simulink model "simulacao_relatorio"  (R2018a)
settings: Solver=VariableStepAuto  StartTime=0.0  StopTime=10000  RelTol=1e-3
undefined symbols (not defined in the file or in its folder): sigbuilder_block
settings Model: Creator=Christopher  LastModifiedBy=Christopher

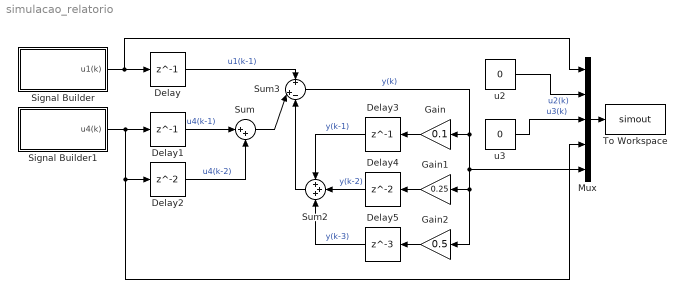
== system simulacao_relatorio ==
  Delay : Delay  DelayLength=1
  Delay1 : Delay  DelayLength=1
  Delay2 : Delay
  Delay3 : Delay  DelayLength=1
  Delay4 : Delay
  Delay5 : Delay  DelayLength=3
  Gain : Gain  Gain=0.1
  Gain1 : Gain  Gain=0.25
  Gain2 : Gain  Gain=0.5
  Mux : Mux  Inputs=5
  Signal Builder : Subsystem  Tag=STV Subsys  LoadFcn=sigbuilder_block('load',[437.6 199.2 550.4 400 ]);  StartFcn=sigbuilder_block('start');  StopFcn=sigbuilder_block('stop');  ClipboardFcn=sigbuilder_block('clipboard');  mask(Sigbuilder block){tuvar=[0:10]}
      mask help: Simulink:masks:SigbuilderBlock_MD
      mask init:
      | if ~strcmp(get_param(bdroot(gcbh),'SimulationStatus'),'stopped') tuvar = sigbuilder_block('maskInit'); end
      settings: CopyFcn=sigbuilder_block('copy');  DeleteFcn=sigbuilder_block('delete');  ModelCloseFcn=sigbuilder_block('modelClose');  PreSaveFcn=sigbuilder_block('preSave');  PauseFcn=sigbuilder_block('pause');  ContinueFcn=sigbuilder_block('continue');  NameChangeFcn=sigbuilder_block('namechange');  OpenFcn=sigbuilder_block('open',[437.6 199.2 550.4 400 ]);  CloseFcn=sigbuilder_block('close');
      mask Display: plot(0, 0, 100, 100,[2, 2, 32, 32, 2], [68, 8, 8, 68, 68],[32, 2], [38, 38], [32, 19, 2],[53, 60, 44], [32, 17, 17, 2],[16, 16, 31, 31]);txt = getActiveGroup(gcbh);text(2, 100, txt,'verticalAlignment', 'top');
  Signal Builder1 : Subsystem  Tag=STV Subsys  LoadFcn=sigbuilder_block('load');  StartFcn=sigbuilder_block('start');  StopFcn=sigbuilder_block('stop');  ClipboardFcn=sigbuilder_block('clipboard');  mask(Sigbuilder block){tuvar=[0:10]}
      mask help: Simulink:masks:SigbuilderBlock_MD
      mask init:
      | if ~strcmp(get_param(bdroot(gcbh),'SimulationStatus'),'stopped') tuvar = sigbuilder_block('maskInit'); end
      settings: CopyFcn=sigbuilder_block('copy');  DeleteFcn=sigbuilder_block('delete');  ModelCloseFcn=sigbuilder_block('modelClose');  PreSaveFcn=sigbuilder_block('preSave');  PauseFcn=sigbuilder_block('pause');  ContinueFcn=sigbuilder_block('continue');  NameChangeFcn=sigbuilder_block('namechange');  OpenFcn=sigbuilder_block('open',[437.6 199.2 550.4 400 ]);  CloseFcn=sigbuilder_block('close');
      mask Display: plot(0, 0, 100, 100,[2, 2, 32, 32, 2], [68, 8, 8, 68, 68],[32, 2], [38, 38], [32, 19, 2],[53, 60, 44], [32, 17, 17, 2],[16, 16, 31, 31]);txt = getActiveGroup(gcbh);text(2, 100, txt,'verticalAlignment', 'top');
  Sum : Sum  Inputs=|++
  Sum2 : Sum  Inputs=+++
  Sum3 : Sum  Inputs=+|+-
  To Workspace : ToWorkspace  VariableName=simout  SampleTime=-1
  u2 : Constant  Value=0  SampleTime=1
  u3 : Constant  Value=0  SampleTime=1
  wires:
  Delay1/1 -> Sum/1  "u4(k-1)"
  Delay2/1 -> Sum/2  "u4(k-2)"
  Delay/1 -> Sum3/1  "u1(k-1)"
  Sum/1 -> Sum3/2
  Sum3/1 -> Gain2/1, Gain1/1, Mux/5, Gain/1  "y(k)"
  Delay3/1 -> Sum2/1  "y(k-1)"
  Delay4/1 -> Sum2/2  "y(k-2)"
  Delay5/1 -> Sum2/3  "y(k-3)"
  Sum2/1 -> Sum3/3
  Mux/1 -> To Workspace/1
  u2/1 -> Mux/2  "u2(k)"
  u3/1 -> Mux/3  "u3(k)"
  Gain/1 -> Delay3/1
  Gain1/1 -> Delay4/1
  Gain2/1 -> Delay5/1
  Signal Builder/1(u1(k)) -> Mux/1, Delay/1
  Signal Builder1/1(u4(k)) -> Mux/4, Delay2/1, Delay1/1

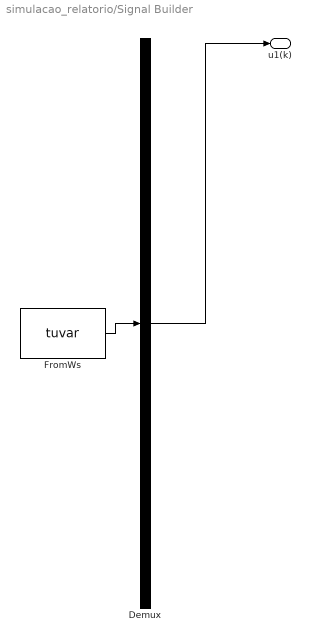
== system simulacao_relatorio/Signal Builder ==
  Demux : Demux  Tag=STV Demux  Outputs=1
  FromWs : FromWorkspace  Tag=STV FromWs  VariableName=tuvar  SampleTime=0
      SigBuilderData=|
      | common.afterFinalStr = 'Extrapolate'
      | common.sampleTime = 0
      | dataSet.timeRange = [0 10]
      | dataSet.name = 'Group 1'
      | sbobj.Groups.Name = 'Group 1'
      | sbobj.Groups.Signals.Name = 'u1(k)'
      | sbobj.Groups.Signals.XData = [0 4 4 6 6 10]
      | sbobj.Groups.Signals.YData = [0 0 1 1 0 0]
  u1(k) : Outport  Tag=STV Outport
  wires:
  Demux/1 -> u1(k)/1
  FromWs/1 -> Demux/1

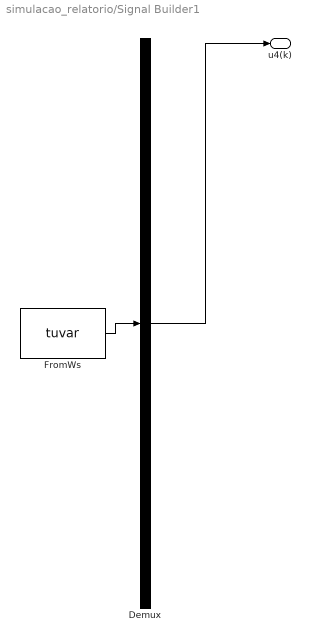
== system simulacao_relatorio/Signal Builder1 ==
  Demux : Demux  Tag=STV Demux  Outputs=1
  FromWs : FromWorkspace  Tag=STV FromWs  VariableName=tuvar  SampleTime=0
      SigBuilderData=|
      | common.afterFinalStr = 'Extrapolate'
      | common.sampleTime = 0
      | dataSet.timeRange = [0 10]
      | dataSet.name = 'Group 2'
      | sbobj.Groups.Name = 'Group 2'
      | sbobj.Groups.Signals.Name = 'u4(k)'
      | sbobj.Groups.Signals.XData = [0 1.8 1.8 6 6 10]
      | sbobj.Groups.Signals.YData = [0 0 1 1 0 0]
  u4(k) : Outport  Tag=STV Outport
  wires:
  Demux/1 -> u4(k)/1
  FromWs/1 -> Demux/1
